simulink model "Wiper_Model"  (R2023a)
settings: Solver=FixedStepAuto  StartTime=0.0  StopTime=inf  FixedStep=0.1  RelTol=1e-3
settings Model: Creator=Abdelateef  LastModifiedBy=Abdelateef

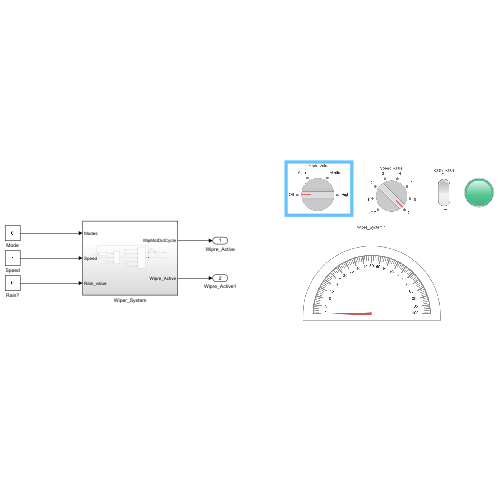
[thumbnail: Simulink's stored preview of the top-level diagram]
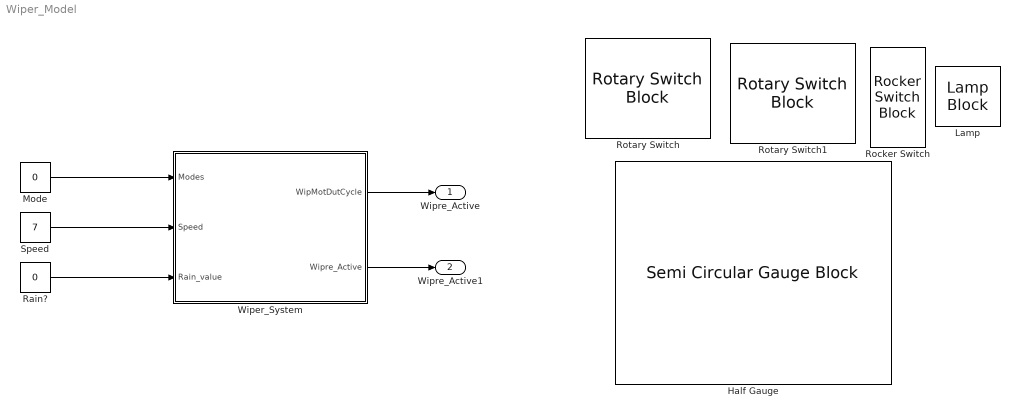
== system Wiper_Model ==
  Half Gauge : SemiCircularGaugeBlock
  Lamp : LampBlock  LabelPosition=Hide
  Mode : Constant  Value=0
  Rain? : Constant  Value=0  OutDataTypeStr=boolean
  Rocker Switch : RockerSwitchBlock
      settings: Values={{'Off', 'On'}, [0 1]}
  Rotary Switch : RotarySwitchBlock
      settings: Values={{'Off', 'Auto', 'Medium', 'High'}, [0 1 2 3]}
  Rotary Switch1 : RotarySwitchBlock
      settings: Values={{'Off', '1', '2', '3', '4', '5', '6', '7'}, [0 1 2 3 4 5 6 7]}
  Speed : Constant  Value=7
  Wiper_System : Subsystem
  Wipre_Active : Outport
  Wipre_Active1 : Outport  Port=2
  wires:
  Mode/1 -> Wiper_System/1(Modes)
  Rain?/1 -> Wiper_System/3(Rain_value)
  Speed/1 -> Wiper_System/2(Speed)
  Wiper_System/1(WipMotDutCycle) -> Wipre_Active/1
  Wiper_System/2(Wipre_Active) -> Wipre_Active1/1

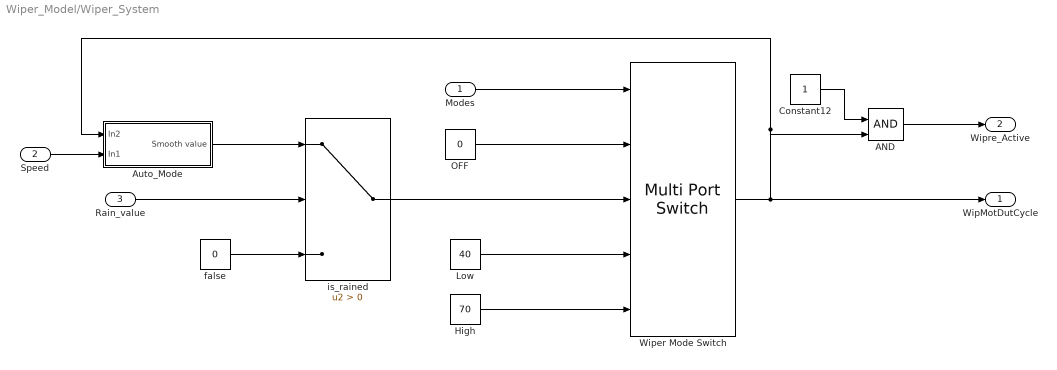
== system Wiper_Model/Wiper_System ==
  Modes : Inport
  Speed : Inport  Port=2
  Rain_value : Inport  Port=3
  AND : Logic  IconShape=distinctive  AllPortsSameDT=off  OutDataTypeStr=boolean
  Auto_Mode : Subsystem
  Constant12 : Constant
  High : Constant  Value=70
  Low : Constant  Value=40
  OFF : Constant  Value=0
  Wiper Mode Switch : MultiPortSwitch  DataPortOrder=Zero-based contiguous  Inputs=4  zeroidx=on  SaturateOnIntegerOverflow=off  InputSameDT=off
  false : Constant  Value=0
  is_rained : Switch  Criteria=u2 > Threshold  SaturateOnIntegerOverflow=off  InputSameDT=off
  WipMotDutCycle : Outport
  Wipre_Active : Outport  Port=2
  wires:
  Modes/1 -> Wiper Mode Switch/1
  OFF/1 -> Wiper Mode Switch/2
  Low/1 -> Wiper Mode Switch/4
  High/1 -> Wiper Mode Switch/5
  Rain_value/1 -> is_rained/2
  is_rained/1 -> Wiper Mode Switch/3
  Constant12/1 -> AND/1
  AND/1 -> Wipre_Active/1
  false/1 -> is_rained/3
  Wiper Mode Switch/1 -> WipMotDutCycle/1, Auto_Mode/1(In2), AND/2
  Speed/1 -> Auto_Mode/2(In1)
  Auto_Mode/1(Smooth value) -> is_rained/1

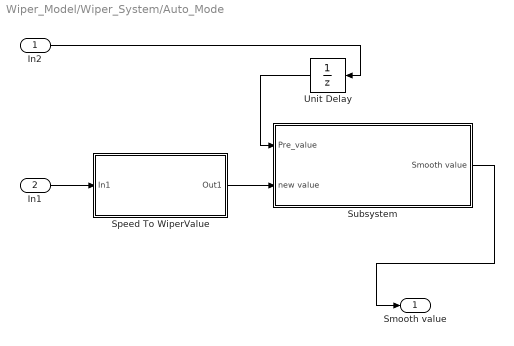
== system Wiper_Model/Wiper_System/Auto_Mode ==
  In2 : Inport
  In1 : Inport  Port=2
  Speed To WiperValue : Subsystem
  Subsystem : Subsystem
  Unit Delay : UnitDelay  SampleTime=-1  HasFrameUpgradeWarning=on
  Smooth value : Outport
  wires:
  Speed To WiperValue/1(Out1) -> Subsystem/2(new value)
  In2/1 -> Unit Delay/1
  Unit Delay/1 -> Subsystem/1(Pre_value)
  In1/1 -> Speed To WiperValue/1(In1)
  Subsystem/1(Smooth value) -> Smooth value/1

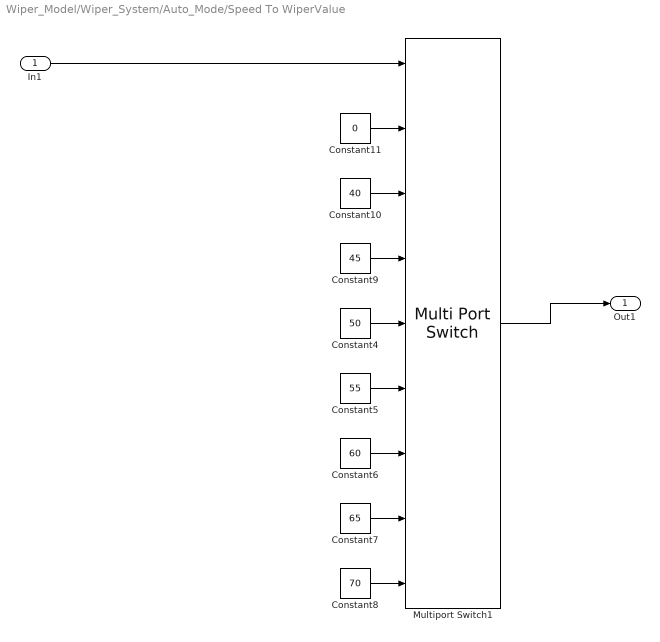
== system Wiper_Model/Wiper_System/Auto_Mode/Speed To WiperValue ==
  In1 : Inport
  Constant10 : Constant  Value=40
  Constant11 : Constant  Value=0
  Constant4 : Constant  Value=50
  Constant5 : Constant  Value=55
  Constant6 : Constant  Value=60
  Constant7 : Constant  Value=65
  Constant8 : Constant  Value=70
  Constant9 : Constant  Value=45
  Multiport Switch1 : MultiPortSwitch  DataPortOrder=Zero-based contiguous  Inputs=8  zeroidx=on  SaturateOnIntegerOverflow=off  InputSameDT=off
  Out1 : Outport
  wires:
  Constant6/1 -> Multiport Switch1/7
  Constant10/1 -> Multiport Switch1/3
  Constant8/1 -> Multiport Switch1/9
  Constant5/1 -> Multiport Switch1/6
  Constant4/1 -> Multiport Switch1/5
  Constant7/1 -> Multiport Switch1/8
  Constant9/1 -> Multiport Switch1/4
  Constant11/1 -> Multiport Switch1/2
  Multiport Switch1/1 -> Out1/1
  In1/1 -> Multiport Switch1/1

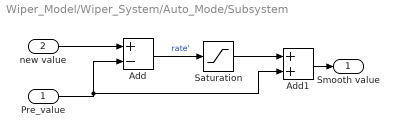
== system Wiper_Model/Wiper_System/Auto_Mode/Subsystem ==
  Pre_value : Inport
  new value : Inport  Port=2
  Add : Sum  Inputs=+-
  Add1 : Sum
  Saturation : Saturate  UpperLimit=0.005  LowerLimit=-0.005
  Smooth value : Outport
  wires:
  Add/1 -> Saturation/1  "rate'"
  Saturation/1 -> Add1/1
  Pre_value/1 -> Add1/2, Add/2
  new value/1 -> Add/1
  Add1/1 -> Smooth value/1
